simulink model "multiplier2"  (R2018b)
settings: Solver=VariableStepAuto  StartTime=0.0  StopTime=10.0  RelTol=1e-3
settings Model: Creator=annat  LastModifiedBy=annat

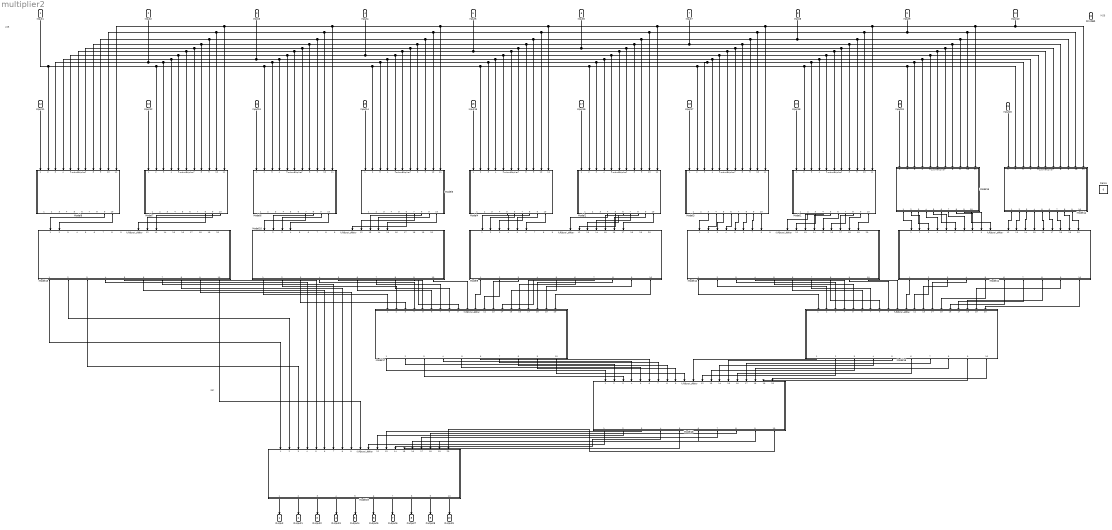
== system multiplier2 ==
  note: 35*
  note: MSB
  note: LSB
  "Input1 " : Inport
  Input2 : Inport  Port=2
  Input3 : Inport  Port=3
  Input4 : Inport  Port=4
  Input5 : Inport  Port=5
  "Input6 " : Inport  Port=6
  Input7 : Inport  Port=7
  Input8 : Inport  Port=8
  Input9 : Inport  Port=9
  Input10 : Inport  Port=10
  DIVIDER : Inport  Port=11
  Input11 : Inport  Port=12
  Input12 : Inport  Port=13
  Input13 : Inport  Port=14
  Input14 : Inport  Port=15
  Input15 : Inport  Port=16
  Input16 : Inport  Port=17
  Input17 : Inport  Port=18
  Input18 : Inport  Port=19
  Input19 : Inport  Port=20
  Input20 : Inport  Port=21
  Model{1..8,14..15} (10 alike) : ModelReference  ModelNameDialog=submultiplier  SimulationMode=Normal  ModelReferenceVersion=1.7
  Model{9..13,16..19} (9 alike) : ModelReference  ModelNameDialog=full_total_adder  SimulationMode=Normal  ModelReferenceVersion=1.4
  Zero1 : Constant  Value=0  OutDataTypeStr=Inherit: Inherit via back propagation
  Output : Outport
  Output1 : Outport  Port=2
  Output2 : Outport  Port=3
  Output3 : Outport  Port=4
  Output4 : Outport  Port=5
  Output5 : Outport  Port=6
  Output6 : Outport  Port=7
  Output7 : Outport  Port=8
  Output8 : Outport  Port=9
  Output9 : Outport  Port=10
  wires:
  Input18/1 -> Model1/1
  Input17/1 -> Model3/1
  Input16/1 -> Model2/1
  Input15/1 -> Model4/1
  Input14/1 -> Model5/1
  Input13/1 -> Model6/1
  Input11/1 -> Model8/1
  Input12/1 -> Model7/1
  "Input1 "/1 -> Model6/2, Model5/2, Model14/2, Model15/2, Model1/2, Model3/2, Model2/2, Model4/2, Model7/2, Model8/2
  Input2/1 -> Model8/3, Model7/3, Model6/3, Model5/3, Model14/3, Model15/3, Model1/3, Model3/3, Model2/3, Model4/3
  Input3/1 -> Model5/4, Model14/4, Model15/4, Model1/4, Model3/4, Model2/4, Model4/4, Model6/4, Model8/4, Model7/4
  Input4/1 -> Model14/5, Model15/5, Model1/5, Model3/5, Model2/5, Model4/5, Model5/5, Model8/5, Model7/5, Model6/5
  Input5/1 -> Model8/6, Model7/6, Model6/6, Model5/6, Model14/6, Model15/6, Model1/6, Model3/6, Model2/6, Model4/6
  "Input6 "/1 -> Model8/7, Model7/7, Model6/7, Model5/7, Model4/7, Model14/7, Model15/7, Model1/7, Model3/7, Model2/7
  Input7/1 -> Model8/8, Model7/8, Model6/8, Model5/8, Model4/8, Model2/8, Model14/8, Model15/8, Model1/8, Model3/8
  Input8/1 -> Model14/9, Model15/9, Model1/9, Model5/9, Model8/9, Model7/9, Model6/9, Model4/9, Model2/9, Model3/9
  Input19/1 -> Model15/1
  Input20/1 -> Model14/1
  Input9/1 -> Model14/10, Model15/10, Model2/10, Model4/10, Model6/10, Model8/10, Model7/10, Model5/10, Model3/10, Model1/10
  Input10/1 -> Model1/11, Model8/11, Model7/11, Model6/11, Model5/11, Model4/11, Model2/11, Model3/11, Model15/11, Model14/11
  Model12/1 -> Model16/1
  Model12/2 -> Model16/2
  Model12/3 -> Model16/3
  Model12/4 -> Model16/4
  Model12/5 -> Model16/5
  Model12/6 -> Model16/6
  Model12/7 -> Model16/7
  Model12/8 -> Model16/8
  Model12/9 -> Model16/9
  Model12/10 -> Model16/10
  Model11/1 -> Model16/11
  Model11/2 -> Model16/12
  Model11/3 -> Model16/13
  Model11/4 -> Model16/14
  Model11/5 -> Model16/15
  Model11/6 -> Model16/16
  Model11/7 -> Model16/17
  Model11/8 -> Model16/18
  Model11/9 -> Model16/19
  Model11/10 -> Model16/20
  Model9/10 -> Model17/20
  Model9/9 -> Model17/19
  Model9/8 -> Model17/18
  Model9/7 -> Model17/17
  Model9/6 -> Model17/16
  Model9/5 -> Model17/15
  Model9/4 -> Model17/14
  Model9/3 -> Model17/13
  Model9/2 -> Model17/12
  Model9/1 -> Model17/11
  Model10/1 -> Model17/1
  Model10/2 -> Model17/2
  Model10/3 -> Model17/3
  Model10/4 -> Model17/4
  Model10/5 -> Model17/5
  Model10/6 -> Model17/6
  Model10/7 -> Model17/7
  Model10/8 -> Model17/8
  Model10/9 -> Model17/9
  Model10/10 -> Model17/10
  Model16/10 -> Model18/20
  Model16/9 -> Model18/19
  Model16/8 -> Model18/18
  Model16/7 -> Model18/17
  Model16/6 -> Model18/16
  Model16/5 -> Model18/15
  Model16/4 -> Model18/14
  Model16/3 -> Model18/13
  Model16/2 -> Model18/12
  Model16/1 -> Model18/11
  Model17/1 -> Model18/1
  Model17/2 -> Model18/2
  Model17/3 -> Model18/3
  Model17/4 -> Model18/4
  Model17/5 -> Model18/5
  Model17/6 -> Model18/6
  Model17/7 -> Model18/7
  Model17/8 -> Model18/8
  Model17/9 -> Model18/9
  Model17/10 -> Model18/10
  Model13/1 -> Model19/1
  Model13/2 -> Model19/2
  Model13/3 -> Model19/3
  Model13/4 -> Model19/4
  Model13/5 -> Model19/5
  Model13/6 -> Model19/6
  Model13/7 -> Model19/7
  Model13/8 -> Model19/8
  Model13/9 -> Model19/9
  Model13/10 -> Model19/10
  Model18/1 -> Model19/11
  Model18/2 -> Model19/12
  Model18/3 -> Model19/13
  Model18/4 -> Model19/14
  Model18/5 -> Model19/15
  Model18/6 -> Model19/16
  Model18/7 -> Model19/17
  Model18/8 -> Model19/18
  Model18/9 -> Model19/19
  Model18/10 -> Model19/20
  Model19/1 -> Output/1
  Model19/2 -> Output1/1
  Model19/3 -> Output2/1
  Model19/4 -> Output3/1
  Model19/5 -> Output4/1
  Model19/6 -> Output5/1
  Model19/7 -> Output6/1
  Model19/8 -> Output7/1
  Model19/9 -> Output8/1
  Model19/10 -> Output9/1
  Model15/1 -> Model11/1
  Model15/2 -> Model11/2
  Model15/3 -> Model11/3
  Model15/4 -> Model11/4
  Model15/5 -> Model11/5
  Model15/6 -> Model11/6
  Model15/7 -> Model11/7
  Model15/8 -> Model11/8
  Model15/9 -> Model11/9
  Model15/10 -> Model11/10
  Model8/10 -> Model13/2
  Model8/9 -> Model13/1
  Model7/8 -> Model13/11
  Model7/9 -> Model13/12
  Model7/10 -> Model13/13
  Model6/10 -> Model10/4
  Model6/9 -> Model10/3
  Model6/8 -> Model10/2
  Model6/7 -> Model10/1
  Model5/10 -> Model10/15
  Model5/9 -> Model10/14
  Model5/8 -> Model10/13
  Model5/7 -> Model10/12
  Model5/6 -> Model10/11
  Model4/10 -> Model9/6
  Model4/9 -> Model9/5
  Model4/8 -> Model9/4
  Model4/7 -> Model9/3
  Model4/6 -> Model9/2
  Model4/5 -> Model9/1
  Model2/10 -> Model9/17
  Model2/9 -> Model9/16
  Model2/8 -> Model9/15
  Model2/7 -> Model9/14
  Model2/6 -> Model9/13
  Model2/5 -> Model9/12
  Model2/4 -> Model9/11
  Model3/10 -> Model12/8
  Model3/9 -> Model12/7
  Model3/8 -> Model12/6
  Model3/7 -> Model12/5
  Model3/6 -> Model12/4
  Model3/5 -> Model12/3
  Model3/4 -> Model12/2
  Model3/3 -> Model12/1
  Model1/10 -> Model12/19
  Model1/9 -> Model12/18
  Model1/8 -> Model12/17
  Model1/7 -> Model12/16
  Model1/6 -> Model12/15
  Model1/5 -> Model12/14
  Model1/4 -> Model12/13
  Model1/3 -> Model12/12
  Model1/2 -> Model12/11
  Model14/9 -> Model11/20
  Model14/8 -> Model11/19
  Model14/7 -> Model11/18
  Model14/6 -> Model11/17
  Model14/5 -> Model11/16
  Model14/4 -> Model11/15
  Model14/3 -> Model11/14
  Model14/2 -> Model11/13
  Model14/1 -> Model11/12
